simulink model "sequentialProcessorNarenKolli"  (R2018b)
settings: Solver=VariableStepAuto  StartTime=0.0  StopTime=10  RelTol=1e-3
libraries: hdlsllib x172, simulink_extras x9
(part 3 of 4)

== system sequentialProcessorNarenKolli/8-Bit_Processor /8-Bit_Multiplier/First 8-Bit_Adder/Full Adder5 ==
  X : Inport
  Y : Inport  Port=2
  Z : Inport  Port=3
  Half Adder : Subsystem
  Half Adder1 : Subsystem
  OR : Logic  Operator=OR  AllPortsSameDT=off  OutDataTypeStr=boolean
  S : Outport
  C : Outport  Port=2
  wires:
  Half Adder/2(Carry) -> OR/2
  OR/1 -> C/1
  Z/1 -> Half Adder1/2(B)
  X/1 -> Half Adder/1(A)
  Half Adder1/1(Sum) -> S/1
  Half Adder/1(Sum) -> Half Adder1/1(A)
  Y/1 -> Half Adder/2(B)
  Half Adder1/2(Carry) -> OR/1

== system sequentialProcessorNarenKolli/8-Bit_Processor /8-Bit_Multiplier/First 8-Bit_Adder/Full Adder6 ==
  X : Inport
  Y : Inport  Port=2
  Z : Inport  Port=3
  Half Adder : Subsystem
  Half Adder1 : Subsystem
  OR : Logic  Operator=OR  AllPortsSameDT=off  OutDataTypeStr=boolean
  S : Outport
  C : Outport  Port=2
  wires:
  Half Adder/2(Carry) -> OR/2
  OR/1 -> C/1
  Z/1 -> Half Adder1/2(B)
  X/1 -> Half Adder/1(A)
  Half Adder1/1(Sum) -> S/1
  Half Adder/1(Sum) -> Half Adder1/1(A)
  Y/1 -> Half Adder/2(B)
  Half Adder1/2(Carry) -> OR/1

== system sequentialProcessorNarenKolli/8-Bit_Processor /8-Bit_Multiplier/First 8-Bit_Adder/Full Adder7 ==
  X : Inport
  Y : Inport  Port=2
  Z : Inport  Port=3
  Half Adder : Subsystem
  Half Adder1 : Subsystem
  OR : Logic  Operator=OR  AllPortsSameDT=off  OutDataTypeStr=boolean
  S : Outport
  C : Outport  Port=2
  wires:
  Half Adder/2(Carry) -> OR/2
  OR/1 -> C/1
  Z/1 -> Half Adder1/2(B)
  X/1 -> Half Adder/1(A)
  Half Adder1/1(Sum) -> S/1
  Half Adder/1(Sum) -> Half Adder1/1(A)
  Y/1 -> Half Adder/2(B)
  Half Adder1/2(Carry) -> OR/1

== system sequentialProcessorNarenKolli/8-Bit_Processor /8-Bit_Multiplier/First 8-Bit_Adder/Slicer ==
  X : Inport  OutDataTypeStr=uint8  SampleTime=1
  Bit Slice : hdlsllib/Logic and Bit Operations/Bit Slice  lidx=7  ridx=7
  Bit Slice1 : hdlsllib/Logic and Bit Operations/Bit Slice  lidx=6  ridx=6
  Bit Slice2 : hdlsllib/Logic and Bit Operations/Bit Slice  lidx=5  ridx=5
  Bit Slice3 : hdlsllib/Logic and Bit Operations/Bit Slice  lidx=4  ridx=4
  Bit Slice4 : hdlsllib/Logic and Bit Operations/Bit Slice  lidx=3  ridx=3
  Bit Slice5 : hdlsllib/Logic and Bit Operations/Bit Slice  lidx=2  ridx=2
  Bit Slice6 : hdlsllib/Logic and Bit Operations/Bit Slice  lidx=1  ridx=1
  Bit Slice7 : hdlsllib/Logic and Bit Operations/Bit Slice  lidx=0  ridx=0
  Data Type Conversion{,1..7} (8 alike) : DataTypeConversion
  Y7 : Outport
  Y6 : Outport  Port=2
  Y5 : Outport  Port=3
  Y4 : Outport  Port=4
  Y3 : Outport  Port=5
  Y2 : Outport  Port=6
  Y1 : Outport  Port=7
  Y0 : Outport  Port=8
  wires:
  Data Type Conversion4/1 -> Y4/1
  Bit Slice3/1 -> Data Type Conversion4/1
  X/1 -> Bit Slice3/1, Bit Slice2/1, Bit Slice1/1, Bit Slice/1, Bit Slice4/1, Bit Slice5/1, Bit Slice6/1, Bit Slice7/1
  Bit Slice1/1 -> Data Type Conversion6/1
  Data Type Conversion1/1 -> Y1/1
  Bit Slice6/1 -> Data Type Conversion1/1
  Bit Slice5/1 -> Data Type Conversion2/1
  Bit Slice2/1 -> Data Type Conversion5/1
  Data Type Conversion/1 -> Y0/1
  Bit Slice4/1 -> Data Type Conversion3/1
  Bit Slice/1 -> Data Type Conversion7/1
  Data Type Conversion7/1 -> Y7/1
  Bit Slice7/1 -> Data Type Conversion/1
  Data Type Conversion3/1 -> Y3/1
  Data Type Conversion5/1 -> Y5/1
  Data Type Conversion6/1 -> Y6/1
  Data Type Conversion2/1 -> Y2/1

== system sequentialProcessorNarenKolli/8-Bit_Processor /8-Bit_Multiplier/First 8-Bit_Adder/Slicer1 ==
  X : Inport  OutDataTypeStr=uint8  SampleTime=1
  Bit Slice : hdlsllib/Logic and Bit Operations/Bit Slice  lidx=7  ridx=7
  Bit Slice1 : hdlsllib/Logic and Bit Operations/Bit Slice  lidx=6  ridx=6
  Bit Slice2 : hdlsllib/Logic and Bit Operations/Bit Slice  lidx=5  ridx=5
  Bit Slice3 : hdlsllib/Logic and Bit Operations/Bit Slice  lidx=4  ridx=4
  Bit Slice4 : hdlsllib/Logic and Bit Operations/Bit Slice  lidx=3  ridx=3
  Bit Slice5 : hdlsllib/Logic and Bit Operations/Bit Slice  lidx=2  ridx=2
  Bit Slice6 : hdlsllib/Logic and Bit Operations/Bit Slice  lidx=1  ridx=1
  Bit Slice7 : hdlsllib/Logic and Bit Operations/Bit Slice  lidx=0  ridx=0
  Data Type Conversion{,1..7} (8 alike) : DataTypeConversion
  Y7 : Outport
  Y6 : Outport  Port=2
  Y5 : Outport  Port=3
  Y4 : Outport  Port=4
  Y3 : Outport  Port=5
  Y2 : Outport  Port=6
  Y1 : Outport  Port=7
  Y0 : Outport  Port=8
  wires:
  Data Type Conversion4/1 -> Y4/1
  Bit Slice3/1 -> Data Type Conversion4/1
  X/1 -> Bit Slice3/1, Bit Slice2/1, Bit Slice1/1, Bit Slice/1, Bit Slice4/1, Bit Slice5/1, Bit Slice6/1, Bit Slice7/1
  Bit Slice1/1 -> Data Type Conversion6/1
  Data Type Conversion1/1 -> Y1/1
  Bit Slice6/1 -> Data Type Conversion1/1
  Bit Slice5/1 -> Data Type Conversion2/1
  Bit Slice2/1 -> Data Type Conversion5/1
  Data Type Conversion/1 -> Y0/1
  Bit Slice4/1 -> Data Type Conversion3/1
  Bit Slice/1 -> Data Type Conversion7/1
  Data Type Conversion7/1 -> Y7/1
  Bit Slice7/1 -> Data Type Conversion/1
  Data Type Conversion3/1 -> Y3/1
  Data Type Conversion5/1 -> Y5/1
  Data Type Conversion6/1 -> Y6/1
  Data Type Conversion2/1 -> Y2/1

== system sequentialProcessorNarenKolli/8-Bit_Processor /8-Bit_Multiplier/Second 4x4 Multiplier/Full Adder ==
  X : Inport
  Y : Inport  Port=2
  Z : Inport  Port=3
  Half Adder : Subsystem
  Half Adder1 : Subsystem
  OR : Logic  Operator=OR  AllPortsSameDT=off  OutDataTypeStr=boolean
  S : Outport
  C : Outport  Port=2
  wires:
  Half Adder/2(Carry) -> OR/2
  OR/1 -> C/1
  Z/1 -> Half Adder1/2(B)
  X/1 -> Half Adder/1(A)
  Half Adder1/1(Sum) -> S/1
  Half Adder/1(Sum) -> Half Adder1/1(A)
  Y/1 -> Half Adder/2(B)
  Half Adder1/2(Carry) -> OR/1

== system sequentialProcessorNarenKolli/8-Bit_Processor /8-Bit_Multiplier/Second 4x4 Multiplier/Full Adder1 ==
  X : Inport
  Y : Inport  Port=2
  Z : Inport  Port=3
  Half Adder : Subsystem
  Half Adder1 : Subsystem
  OR : Logic  Operator=OR  AllPortsSameDT=off  OutDataTypeStr=boolean
  S : Outport
  C : Outport  Port=2
  wires:
  Half Adder/2(Carry) -> OR/2
  OR/1 -> C/1
  Z/1 -> Half Adder1/2(B)
  X/1 -> Half Adder/1(A)
  Half Adder1/1(Sum) -> S/1
  Half Adder/1(Sum) -> Half Adder1/1(A)
  Y/1 -> Half Adder/2(B)
  Half Adder1/2(Carry) -> OR/1

== system sequentialProcessorNarenKolli/8-Bit_Processor /8-Bit_Multiplier/Second 4x4 Multiplier/Full Adder2 ==
  X : Inport
  Y : Inport  Port=2
  Z : Inport  Port=3
  Half Adder : Subsystem
  Half Adder1 : Subsystem
  OR : Logic  Operator=OR  AllPortsSameDT=off  OutDataTypeStr=boolean
  S : Outport
  C : Outport  Port=2
  wires:
  Half Adder/2(Carry) -> OR/2
  OR/1 -> C/1
  Z/1 -> Half Adder1/2(B)
  X/1 -> Half Adder/1(A)
  Half Adder1/1(Sum) -> S/1
  Half Adder/1(Sum) -> Half Adder1/1(A)
  Y/1 -> Half Adder/2(B)
  Half Adder1/2(Carry) -> OR/1

== system sequentialProcessorNarenKolli/8-Bit_Processor /8-Bit_Multiplier/Second 4x4 Multiplier/Full Adder3 ==
  X : Inport
  Y : Inport  Port=2
  Z : Inport  Port=3
  Half Adder : Subsystem
  Half Adder1 : Subsystem
  OR : Logic  Operator=OR  AllPortsSameDT=off  OutDataTypeStr=boolean
  S : Outport
  C : Outport  Port=2
  wires:
  Half Adder/2(Carry) -> OR/2
  OR/1 -> C/1
  Z/1 -> Half Adder1/2(B)
  X/1 -> Half Adder/1(A)
  Half Adder1/1(Sum) -> S/1
  Half Adder/1(Sum) -> Half Adder1/1(A)
  Y/1 -> Half Adder/2(B)
  Half Adder1/2(Carry) -> OR/1

== system sequentialProcessorNarenKolli/8-Bit_Processor /8-Bit_Multiplier/Second 4x4 Multiplier/Full Adder4 ==
  X : Inport
  Y : Inport  Port=2
  Z : Inport  Port=3
  Half Adder : Subsystem
  Half Adder1 : Subsystem
  OR : Logic  Operator=OR  AllPortsSameDT=off  OutDataTypeStr=boolean
  S : Outport
  C : Outport  Port=2
  wires:
  Half Adder/2(Carry) -> OR/2
  OR/1 -> C/1
  Z/1 -> Half Adder1/2(B)
  X/1 -> Half Adder/1(A)
  Half Adder1/1(Sum) -> S/1
  Half Adder/1(Sum) -> Half Adder1/1(A)
  Y/1 -> Half Adder/2(B)
  Half Adder1/2(Carry) -> OR/1

== system sequentialProcessorNarenKolli/8-Bit_Processor /8-Bit_Multiplier/Second 4x4 Multiplier/Full Adder5 ==
  X : Inport
  Y : Inport  Port=2
  Z : Inport  Port=3
  Half Adder : Subsystem
  Half Adder1 : Subsystem
  OR : Logic  Operator=OR  AllPortsSameDT=off  OutDataTypeStr=boolean
  S : Outport
  C : Outport  Port=2
  wires:
  Half Adder/2(Carry) -> OR/2
  OR/1 -> C/1
  Z/1 -> Half Adder1/2(B)
  X/1 -> Half Adder/1(A)
  Half Adder1/1(Sum) -> S/1
  Half Adder/1(Sum) -> Half Adder1/1(A)
  Y/1 -> Half Adder/2(B)
  Half Adder1/2(Carry) -> OR/1

== system sequentialProcessorNarenKolli/8-Bit_Processor /8-Bit_Multiplier/Second 4x4 Multiplier/Full Adder6 ==
  X : Inport
  Y : Inport  Port=2
  Z : Inport  Port=3
  Half Adder : Subsystem
  Half Adder1 : Subsystem
  OR : Logic  Operator=OR  AllPortsSameDT=off  OutDataTypeStr=boolean
  S : Outport
  C : Outport  Port=2
  wires:
  Half Adder/2(Carry) -> OR/2
  OR/1 -> C/1
  Z/1 -> Half Adder1/2(B)
  X/1 -> Half Adder/1(A)
  Half Adder1/1(Sum) -> S/1
  Half Adder/1(Sum) -> Half Adder1/1(A)
  Y/1 -> Half Adder/2(B)
  Half Adder1/2(Carry) -> OR/1

== system sequentialProcessorNarenKolli/8-Bit_Processor /8-Bit_Multiplier/Second 4x4 Multiplier/Full Adder7 ==
  X : Inport
  Y : Inport  Port=2
  Z : Inport  Port=3
  Half Adder : Subsystem
  Half Adder1 : Subsystem
  OR : Logic  Operator=OR  AllPortsSameDT=off  OutDataTypeStr=boolean
  S : Outport
  C : Outport  Port=2
  wires:
  Half Adder/2(Carry) -> OR/2
  OR/1 -> C/1
  Z/1 -> Half Adder1/2(B)
  X/1 -> Half Adder/1(A)
  Half Adder1/1(Sum) -> S/1
  Half Adder/1(Sum) -> Half Adder1/1(A)
  Y/1 -> Half Adder/2(B)
  Half Adder1/2(Carry) -> OR/1

== system sequentialProcessorNarenKolli/8-Bit_Processor /8-Bit_Multiplier/Second 4x4 Multiplier/Half Adder ==
  A : Inport
  B : Inport  Port=2
  AND (calculates carry) : Logic  AllPortsSameDT=off  OutDataTypeStr=boolean
  XOR (calculates sum) : Logic  Operator=XOR  AllPortsSameDT=off  OutDataTypeStr=boolean
  Sum : Outport
  Carry : Outport  Port=2
  wires:
  XOR (calculates sum)/1 -> Sum/1
  B/1 -> XOR (calculates sum)/2, AND (calculates carry)/2
  A/1 -> AND (calculates carry)/1, XOR (calculates sum)/1
  AND (calculates carry)/1 -> Carry/1

== system sequentialProcessorNarenKolli/8-Bit_Processor /8-Bit_Multiplier/Second 4x4 Multiplier/Half Adder1 ==
  A : Inport
  B : Inport  Port=2
  AND (calculates carry) : Logic  AllPortsSameDT=off  OutDataTypeStr=boolean
  XOR (calculates sum) : Logic  Operator=XOR  AllPortsSameDT=off  OutDataTypeStr=boolean
  Sum : Outport
  Carry : Outport  Port=2
  wires:
  XOR (calculates sum)/1 -> Sum/1
  B/1 -> XOR (calculates sum)/2, AND (calculates carry)/2
  A/1 -> AND (calculates carry)/1, XOR (calculates sum)/1
  AND (calculates carry)/1 -> Carry/1

== system sequentialProcessorNarenKolli/8-Bit_Processor /8-Bit_Multiplier/Second 4x4 Multiplier/Half Adder2 ==
  A : Inport
  B : Inport  Port=2
  AND (calculates carry) : Logic  AllPortsSameDT=off  OutDataTypeStr=boolean
  XOR (calculates sum) : Logic  Operator=XOR  AllPortsSameDT=off  OutDataTypeStr=boolean
  Sum : Outport
  Carry : Outport  Port=2
  wires:
  XOR (calculates sum)/1 -> Sum/1
  B/1 -> XOR (calculates sum)/2, AND (calculates carry)/2
  A/1 -> AND (calculates carry)/1, XOR (calculates sum)/1
  AND (calculates carry)/1 -> Carry/1

== system sequentialProcessorNarenKolli/8-Bit_Processor /8-Bit_Multiplier/Second 4x4 Multiplier/Half Adder3 ==
  A : Inport
  B : Inport  Port=2
  AND (calculates carry) : Logic  AllPortsSameDT=off  OutDataTypeStr=boolean
  XOR (calculates sum) : Logic  Operator=XOR  AllPortsSameDT=off  OutDataTypeStr=boolean
  Sum : Outport
  Carry : Outport  Port=2
  wires:
  XOR (calculates sum)/1 -> Sum/1
  B/1 -> XOR (calculates sum)/2, AND (calculates carry)/2
  A/1 -> AND (calculates carry)/1, XOR (calculates sum)/1
  AND (calculates carry)/1 -> Carry/1

== system sequentialProcessorNarenKolli/8-Bit_Processor /8-Bit_Multiplier/Second 8-Bit_Adder1/Full Adder ==
  X : Inport
  Y : Inport  Port=2
  Z : Inport  Port=3
  Half Adder : Subsystem
  Half Adder1 : Subsystem
  OR : Logic  Operator=OR  AllPortsSameDT=off  OutDataTypeStr=boolean
  S : Outport
  C : Outport  Port=2
  wires:
  Half Adder/2(Carry) -> OR/2
  OR/1 -> C/1
  Z/1 -> Half Adder1/2(B)
  X/1 -> Half Adder/1(A)
  Half Adder1/1(Sum) -> S/1
  Half Adder/1(Sum) -> Half Adder1/1(A)
  Y/1 -> Half Adder/2(B)
  Half Adder1/2(Carry) -> OR/1

== system sequentialProcessorNarenKolli/8-Bit_Processor /8-Bit_Multiplier/Second 8-Bit_Adder1/Full Adder1 ==
  X : Inport
  Y : Inport  Port=2
  Z : Inport  Port=3
  Half Adder : Subsystem
  Half Adder1 : Subsystem
  OR : Logic  Operator=OR  AllPortsSameDT=off  OutDataTypeStr=boolean
  S : Outport
  C : Outport  Port=2
  wires:
  Half Adder/2(Carry) -> OR/2
  OR/1 -> C/1
  Z/1 -> Half Adder1/2(B)
  X/1 -> Half Adder/1(A)
  Half Adder1/1(Sum) -> S/1
  Half Adder/1(Sum) -> Half Adder1/1(A)
  Y/1 -> Half Adder/2(B)
  Half Adder1/2(Carry) -> OR/1

== system sequentialProcessorNarenKolli/8-Bit_Processor /8-Bit_Multiplier/Second 8-Bit_Adder1/Full Adder2 ==
  X : Inport
  Y : Inport  Port=2
  Z : Inport  Port=3
  Half Adder : Subsystem
  Half Adder1 : Subsystem
  OR : Logic  Operator=OR  AllPortsSameDT=off  OutDataTypeStr=boolean
  S : Outport
  C : Outport  Port=2
  wires:
  Half Adder/2(Carry) -> OR/2
  OR/1 -> C/1
  Z/1 -> Half Adder1/2(B)
  X/1 -> Half Adder/1(A)
  Half Adder1/1(Sum) -> S/1
  Half Adder/1(Sum) -> Half Adder1/1(A)
  Y/1 -> Half Adder/2(B)
  Half Adder1/2(Carry) -> OR/1

== system sequentialProcessorNarenKolli/8-Bit_Processor /8-Bit_Multiplier/Second 8-Bit_Adder1/Full Adder3 ==
  X : Inport
  Y : Inport  Port=2
  Z : Inport  Port=3
  Half Adder : Subsystem
  Half Adder1 : Subsystem
  OR : Logic  Operator=OR  AllPortsSameDT=off  OutDataTypeStr=boolean
  S : Outport
  C : Outport  Port=2
  wires:
  Half Adder/2(Carry) -> OR/2
  OR/1 -> C/1
  Z/1 -> Half Adder1/2(B)
  X/1 -> Half Adder/1(A)
  Half Adder1/1(Sum) -> S/1
  Half Adder/1(Sum) -> Half Adder1/1(A)
  Y/1 -> Half Adder/2(B)
  Half Adder1/2(Carry) -> OR/1

== system sequentialProcessorNarenKolli/8-Bit_Processor /8-Bit_Multiplier/Second 8-Bit_Adder1/Full Adder4 ==
  X : Inport
  Y : Inport  Port=2
  Z : Inport  Port=3
  Half Adder : Subsystem
  Half Adder1 : Subsystem
  OR : Logic  Operator=OR  AllPortsSameDT=off  OutDataTypeStr=boolean
  S : Outport
  C : Outport  Port=2
  wires:
  Half Adder/2(Carry) -> OR/2
  OR/1 -> C/1
  Z/1 -> Half Adder1/2(B)
  X/1 -> Half Adder/1(A)
  Half Adder1/1(Sum) -> S/1
  Half Adder/1(Sum) -> Half Adder1/1(A)
  Y/1 -> Half Adder/2(B)
  Half Adder1/2(Carry) -> OR/1

== system sequentialProcessorNarenKolli/8-Bit_Processor /8-Bit_Multiplier/Second 8-Bit_Adder1/Full Adder5 ==
  X : Inport
  Y : Inport  Port=2
  Z : Inport  Port=3
  Half Adder : Subsystem
  Half Adder1 : Subsystem
  OR : Logic  Operator=OR  AllPortsSameDT=off  OutDataTypeStr=boolean
  S : Outport
  C : Outport  Port=2
  wires:
  Half Adder/2(Carry) -> OR/2
  OR/1 -> C/1
  Z/1 -> Half Adder1/2(B)
  X/1 -> Half Adder/1(A)
  Half Adder1/1(Sum) -> S/1
  Half Adder/1(Sum) -> Half Adder1/1(A)
  Y/1 -> Half Adder/2(B)
  Half Adder1/2(Carry) -> OR/1

== system sequentialProcessorNarenKolli/8-Bit_Processor /8-Bit_Multiplier/Second 8-Bit_Adder1/Full Adder6 ==
  X : Inport
  Y : Inport  Port=2
  Z : Inport  Port=3
  Half Adder : Subsystem
  Half Adder1 : Subsystem
  OR : Logic  Operator=OR  AllPortsSameDT=off  OutDataTypeStr=boolean
  S : Outport
  C : Outport  Port=2
  wires:
  Half Adder/2(Carry) -> OR/2
  OR/1 -> C/1
  Z/1 -> Half Adder1/2(B)
  X/1 -> Half Adder/1(A)
  Half Adder1/1(Sum) -> S/1
  Half Adder/1(Sum) -> Half Adder1/1(A)
  Y/1 -> Half Adder/2(B)
  Half Adder1/2(Carry) -> OR/1

== system sequentialProcessorNarenKolli/8-Bit_Processor /8-Bit_Multiplier/Second 8-Bit_Adder1/Full Adder7 ==
  X : Inport
  Y : Inport  Port=2
  Z : Inport  Port=3
  Half Adder : Subsystem
  Half Adder1 : Subsystem
  OR : Logic  Operator=OR  AllPortsSameDT=off  OutDataTypeStr=boolean
  S : Outport
  C : Outport  Port=2
  wires:
  Half Adder/2(Carry) -> OR/2
  OR/1 -> C/1
  Z/1 -> Half Adder1/2(B)
  X/1 -> Half Adder/1(A)
  Half Adder1/1(Sum) -> S/1
  Half Adder/1(Sum) -> Half Adder1/1(A)
  Y/1 -> Half Adder/2(B)
  Half Adder1/2(Carry) -> OR/1

== system sequentialProcessorNarenKolli/8-Bit_Processor /8-Bit_Multiplier/Second 8-Bit_Adder1/Slicer ==
  X : Inport  OutDataTypeStr=uint8  SampleTime=1
  Bit Slice : hdlsllib/Logic and Bit Operations/Bit Slice  lidx=7  ridx=7
  Bit Slice1 : hdlsllib/Logic and Bit Operations/Bit Slice  lidx=6  ridx=6
  Bit Slice2 : hdlsllib/Logic and Bit Operations/Bit Slice  lidx=5  ridx=5
  Bit Slice3 : hdlsllib/Logic and Bit Operations/Bit Slice  lidx=4  ridx=4
  Bit Slice4 : hdlsllib/Logic and Bit Operations/Bit Slice  lidx=3  ridx=3
  Bit Slice5 : hdlsllib/Logic and Bit Operations/Bit Slice  lidx=2  ridx=2
  Bit Slice6 : hdlsllib/Logic and Bit Operations/Bit Slice  lidx=1  ridx=1
  Bit Slice7 : hdlsllib/Logic and Bit Operations/Bit Slice  lidx=0  ridx=0
  Data Type Conversion{,1..7} (8 alike) : DataTypeConversion
  Y7 : Outport
  Y6 : Outport  Port=2
  Y5 : Outport  Port=3
  Y4 : Outport  Port=4
  Y3 : Outport  Port=5
  Y2 : Outport  Port=6
  Y1 : Outport  Port=7
  Y0 : Outport  Port=8
  wires:
  Data Type Conversion4/1 -> Y4/1
  Bit Slice3/1 -> Data Type Conversion4/1
  X/1 -> Bit Slice3/1, Bit Slice2/1, Bit Slice1/1, Bit Slice/1, Bit Slice4/1, Bit Slice5/1, Bit Slice6/1, Bit Slice7/1
  Bit Slice1/1 -> Data Type Conversion6/1
  Data Type Conversion1/1 -> Y1/1
  Bit Slice6/1 -> Data Type Conversion1/1
  Bit Slice5/1 -> Data Type Conversion2/1
  Bit Slice2/1 -> Data Type Conversion5/1
  Data Type Conversion/1 -> Y0/1
  Bit Slice4/1 -> Data Type Conversion3/1
  Bit Slice/1 -> Data Type Conversion7/1
  Data Type Conversion7/1 -> Y7/1
  Bit Slice7/1 -> Data Type Conversion/1
  Data Type Conversion3/1 -> Y3/1
  Data Type Conversion5/1 -> Y5/1
  Data Type Conversion6/1 -> Y6/1
  Data Type Conversion2/1 -> Y2/1

== system sequentialProcessorNarenKolli/8-Bit_Processor /8-Bit_Multiplier/Second 8-Bit_Adder1/Slicer1 ==
  X : Inport  OutDataTypeStr=uint8  SampleTime=1
  Bit Slice : hdlsllib/Logic and Bit Operations/Bit Slice  lidx=7  ridx=7
  Bit Slice1 : hdlsllib/Logic and Bit Operations/Bit Slice  lidx=6  ridx=6
  Bit Slice2 : hdlsllib/Logic and Bit Operations/Bit Slice  lidx=5  ridx=5
  Bit Slice3 : hdlsllib/Logic and Bit Operations/Bit Slice  lidx=4  ridx=4
  Bit Slice4 : hdlsllib/Logic and Bit Operations/Bit Slice  lidx=3  ridx=3
  Bit Slice5 : hdlsllib/Logic and Bit Operations/Bit Slice  lidx=2  ridx=2
  Bit Slice6 : hdlsllib/Logic and Bit Operations/Bit Slice  lidx=1  ridx=1
  Bit Slice7 : hdlsllib/Logic and Bit Operations/Bit Slice  lidx=0  ridx=0
  Data Type Conversion{,1..7} (8 alike) : DataTypeConversion
  Y7 : Outport
  Y6 : Outport  Port=2
  Y5 : Outport  Port=3
  Y4 : Outport  Port=4
  Y3 : Outport  Port=5
  Y2 : Outport  Port=6
  Y1 : Outport  Port=7
  Y0 : Outport  Port=8
  wires:
  Data Type Conversion4/1 -> Y4/1
  Bit Slice3/1 -> Data Type Conversion4/1
  X/1 -> Bit Slice3/1, Bit Slice2/1, Bit Slice1/1, Bit Slice/1, Bit Slice4/1, Bit Slice5/1, Bit Slice6/1, Bit Slice7/1
  Bit Slice1/1 -> Data Type Conversion6/1
  Data Type Conversion1/1 -> Y1/1
  Bit Slice6/1 -> Data Type Conversion1/1
  Bit Slice5/1 -> Data Type Conversion2/1
  Bit Slice2/1 -> Data Type Conversion5/1
  Data Type Conversion/1 -> Y0/1
  Bit Slice4/1 -> Data Type Conversion3/1
  Bit Slice/1 -> Data Type Conversion7/1
  Data Type Conversion7/1 -> Y7/1
  Bit Slice7/1 -> Data Type Conversion/1
  Data Type Conversion3/1 -> Y3/1
  Data Type Conversion5/1 -> Y5/1
  Data Type Conversion6/1 -> Y6/1
  Data Type Conversion2/1 -> Y2/1

== system sequentialProcessorNarenKolli/8-Bit_Processor /8-Bit_Multiplier/Third 4x4 Multiplier/Full Adder ==
  X : Inport
  Y : Inport  Port=2
  Z : Inport  Port=3
  Half Adder : Subsystem
  Half Adder1 : Subsystem
  OR : Logic  Operator=OR  AllPortsSameDT=off  OutDataTypeStr=boolean
  S : Outport
  C : Outport  Port=2
  wires:
  Half Adder/2(Carry) -> OR/2
  OR/1 -> C/1
  Z/1 -> Half Adder1/2(B)
  X/1 -> Half Adder/1(A)
  Half Adder1/1(Sum) -> S/1
  Half Adder/1(Sum) -> Half Adder1/1(A)
  Y/1 -> Half Adder/2(B)
  Half Adder1/2(Carry) -> OR/1

== system sequentialProcessorNarenKolli/8-Bit_Processor /8-Bit_Multiplier/Third 4x4 Multiplier/Full Adder1 ==
  X : Inport
  Y : Inport  Port=2
  Z : Inport  Port=3
  Half Adder : Subsystem
  Half Adder1 : Subsystem
  OR : Logic  Operator=OR  AllPortsSameDT=off  OutDataTypeStr=boolean
  S : Outport
  C : Outport  Port=2
  wires:
  Half Adder/2(Carry) -> OR/2
  OR/1 -> C/1
  Z/1 -> Half Adder1/2(B)
  X/1 -> Half Adder/1(A)
  Half Adder1/1(Sum) -> S/1
  Half Adder/1(Sum) -> Half Adder1/1(A)
  Y/1 -> Half Adder/2(B)
  Half Adder1/2(Carry) -> OR/1

== system sequentialProcessorNarenKolli/8-Bit_Processor /8-Bit_Multiplier/Third 4x4 Multiplier/Full Adder2 ==
  X : Inport
  Y : Inport  Port=2
  Z : Inport  Port=3
  Half Adder : Subsystem
  Half Adder1 : Subsystem
  OR : Logic  Operator=OR  AllPortsSameDT=off  OutDataTypeStr=boolean
  S : Outport
  C : Outport  Port=2
  wires:
  Half Adder/2(Carry) -> OR/2
  OR/1 -> C/1
  Z/1 -> Half Adder1/2(B)
  X/1 -> Half Adder/1(A)
  Half Adder1/1(Sum) -> S/1
  Half Adder/1(Sum) -> Half Adder1/1(A)
  Y/1 -> Half Adder/2(B)
  Half Adder1/2(Carry) -> OR/1

== system sequentialProcessorNarenKolli/8-Bit_Processor /8-Bit_Multiplier/Third 4x4 Multiplier/Full Adder3 ==
  X : Inport
  Y : Inport  Port=2
  Z : Inport  Port=3
  Half Adder : Subsystem
  Half Adder1 : Subsystem
  OR : Logic  Operator=OR  AllPortsSameDT=off  OutDataTypeStr=boolean
  S : Outport
  C : Outport  Port=2
  wires:
  Half Adder/2(Carry) -> OR/2
  OR/1 -> C/1
  Z/1 -> Half Adder1/2(B)
  X/1 -> Half Adder/1(A)
  Half Adder1/1(Sum) -> S/1
  Half Adder/1(Sum) -> Half Adder1/1(A)
  Y/1 -> Half Adder/2(B)
  Half Adder1/2(Carry) -> OR/1

== system sequentialProcessorNarenKolli/8-Bit_Processor /8-Bit_Multiplier/Third 4x4 Multiplier/Full Adder4 ==
  X : Inport
  Y : Inport  Port=2
  Z : Inport  Port=3
  Half Adder : Subsystem
  Half Adder1 : Subsystem
  OR : Logic  Operator=OR  AllPortsSameDT=off  OutDataTypeStr=boolean
  S : Outport
  C : Outport  Port=2
  wires:
  Half Adder/2(Carry) -> OR/2
  OR/1 -> C/1
  Z/1 -> Half Adder1/2(B)
  X/1 -> Half Adder/1(A)
  Half Adder1/1(Sum) -> S/1
  Half Adder/1(Sum) -> Half Adder1/1(A)
  Y/1 -> Half Adder/2(B)
  Half Adder1/2(Carry) -> OR/1

== system sequentialProcessorNarenKolli/8-Bit_Processor /8-Bit_Multiplier/Third 4x4 Multiplier/Full Adder5 ==
  X : Inport
  Y : Inport  Port=2
  Z : Inport  Port=3
  Half Adder : Subsystem
  Half Adder1 : Subsystem
  OR : Logic  Operator=OR  AllPortsSameDT=off  OutDataTypeStr=boolean
  S : Outport
  C : Outport  Port=2
  wires:
  Half Adder/2(Carry) -> OR/2
  OR/1 -> C/1
  Z/1 -> Half Adder1/2(B)
  X/1 -> Half Adder/1(A)
  Half Adder1/1(Sum) -> S/1
  Half Adder/1(Sum) -> Half Adder1/1(A)
  Y/1 -> Half Adder/2(B)
  Half Adder1/2(Carry) -> OR/1

== system sequentialProcessorNarenKolli/8-Bit_Processor /8-Bit_Multiplier/Third 4x4 Multiplier/Full Adder6 ==
  X : Inport
  Y : Inport  Port=2
  Z : Inport  Port=3
  Half Adder : Subsystem
  Half Adder1 : Subsystem
  OR : Logic  Operator=OR  AllPortsSameDT=off  OutDataTypeStr=boolean
  S : Outport
  C : Outport  Port=2
  wires:
  Half Adder/2(Carry) -> OR/2
  OR/1 -> C/1
  Z/1 -> Half Adder1/2(B)
  X/1 -> Half Adder/1(A)
  Half Adder1/1(Sum) -> S/1
  Half Adder/1(Sum) -> Half Adder1/1(A)
  Y/1 -> Half Adder/2(B)
  Half Adder1/2(Carry) -> OR/1

== system sequentialProcessorNarenKolli/8-Bit_Processor /8-Bit_Multiplier/Third 4x4 Multiplier/Full Adder7 ==
  X : Inport
  Y : Inport  Port=2
  Z : Inport  Port=3
  Half Adder : Subsystem
  Half Adder1 : Subsystem
  OR : Logic  Operator=OR  AllPortsSameDT=off  OutDataTypeStr=boolean
  S : Outport
  C : Outport  Port=2
  wires:
  Half Adder/2(Carry) -> OR/2
  OR/1 -> C/1
  Z/1 -> Half Adder1/2(B)
  X/1 -> Half Adder/1(A)
  Half Adder1/1(Sum) -> S/1
  Half Adder/1(Sum) -> Half Adder1/1(A)
  Y/1 -> Half Adder/2(B)
  Half Adder1/2(Carry) -> OR/1

== system sequentialProcessorNarenKolli/8-Bit_Processor /8-Bit_Multiplier/Third 4x4 Multiplier/Half Adder ==
  A : Inport
  B : Inport  Port=2
  AND (calculates carry) : Logic  AllPortsSameDT=off  OutDataTypeStr=boolean
  XOR (calculates sum) : Logic  Operator=XOR  AllPortsSameDT=off  OutDataTypeStr=boolean
  Sum : Outport
  Carry : Outport  Port=2
  wires:
  XOR (calculates sum)/1 -> Sum/1
  B/1 -> XOR (calculates sum)/2, AND (calculates carry)/2
  A/1 -> AND (calculates carry)/1, XOR (calculates sum)/1
  AND (calculates carry)/1 -> Carry/1

== system sequentialProcessorNarenKolli/8-Bit_Processor /8-Bit_Multiplier/Third 4x4 Multiplier/Half Adder1 ==
  A : Inport
  B : Inport  Port=2
  AND (calculates carry) : Logic  AllPortsSameDT=off  OutDataTypeStr=boolean
  XOR (calculates sum) : Logic  Operator=XOR  AllPortsSameDT=off  OutDataTypeStr=boolean
  Sum : Outport
  Carry : Outport  Port=2
  wires:
  XOR (calculates sum)/1 -> Sum/1
  B/1 -> XOR (calculates sum)/2, AND (calculates carry)/2
  A/1 -> AND (calculates carry)/1, XOR (calculates sum)/1
  AND (calculates carry)/1 -> Carry/1

== system sequentialProcessorNarenKolli/8-Bit_Processor /8-Bit_Multiplier/Third 4x4 Multiplier/Half Adder2 ==
  A : Inport
  B : Inport  Port=2
  AND (calculates carry) : Logic  AllPortsSameDT=off  OutDataTypeStr=boolean
  XOR (calculates sum) : Logic  Operator=XOR  AllPortsSameDT=off  OutDataTypeStr=boolean
  Sum : Outport
  Carry : Outport  Port=2
  wires:
  XOR (calculates sum)/1 -> Sum/1
  B/1 -> XOR (calculates sum)/2, AND (calculates carry)/2
  A/1 -> AND (calculates carry)/1, XOR (calculates sum)/1
  AND (calculates carry)/1 -> Carry/1

== system sequentialProcessorNarenKolli/8-Bit_Processor /8-Bit_Multiplier/Third 4x4 Multiplier/Half Adder3 ==
  A : Inport
  B : Inport  Port=2
  AND (calculates carry) : Logic  AllPortsSameDT=off  OutDataTypeStr=boolean
  XOR (calculates sum) : Logic  Operator=XOR  AllPortsSameDT=off  OutDataTypeStr=boolean
  Sum : Outport
  Carry : Outport  Port=2
  wires:
  XOR (calculates sum)/1 -> Sum/1
  B/1 -> XOR (calculates sum)/2, AND (calculates carry)/2
  A/1 -> AND (calculates carry)/1, XOR (calculates sum)/1
  AND (calculates carry)/1 -> Carry/1

== system sequentialProcessorNarenKolli/8-Bit_Processor /8-Bit_Subtractor/Full Adder 0/Half Adder ==
  A : Inport
  B : Inport  Port=2
  AND (calculates carry) : Logic  AllPortsSameDT=off  OutDataTypeStr=boolean
  XOR (calculates sum) : Logic  Operator=XOR  AllPortsSameDT=off  OutDataTypeStr=boolean
  Sum : Outport
  Carry : Outport  Port=2
  wires:
  XOR (calculates sum)/1 -> Sum/1
  B/1 -> XOR (calculates sum)/2, AND (calculates carry)/2
  A/1 -> AND (calculates carry)/1, XOR (calculates sum)/1
  AND (calculates carry)/1 -> Carry/1

== system sequentialProcessorNarenKolli/8-Bit_Processor /8-Bit_Subtractor/Full Adder 0/Half Adder1 ==
  A : Inport
  B : Inport  Port=2
  AND (calculates carry) : Logic  AllPortsSameDT=off  OutDataTypeStr=boolean
  XOR (calculates sum) : Logic  Operator=XOR  AllPortsSameDT=off  OutDataTypeStr=boolean
  Sum : Outport
  Carry : Outport  Port=2
  wires:
  XOR (calculates sum)/1 -> Sum/1
  B/1 -> XOR (calculates sum)/2, AND (calculates carry)/2
  A/1 -> AND (calculates carry)/1, XOR (calculates sum)/1
  AND (calculates carry)/1 -> Carry/1

== system sequentialProcessorNarenKolli/8-Bit_Processor /8-Bit_Subtractor/Full Adder 1/Half Adder ==
  A : Inport
  B : Inport  Port=2
  AND (calculates carry) : Logic  AllPortsSameDT=off  OutDataTypeStr=boolean
  XOR (calculates sum) : Logic  Operator=XOR  AllPortsSameDT=off  OutDataTypeStr=boolean
  Sum : Outport
  Carry : Outport  Port=2
  wires:
  XOR (calculates sum)/1 -> Sum/1
  B/1 -> XOR (calculates sum)/2, AND (calculates carry)/2
  A/1 -> AND (calculates carry)/1, XOR (calculates sum)/1
  AND (calculates carry)/1 -> Carry/1

== system sequentialProcessorNarenKolli/8-Bit_Processor /8-Bit_Subtractor/Full Adder 1/Half Adder1 ==
  A : Inport
  B : Inport  Port=2
  AND (calculates carry) : Logic  AllPortsSameDT=off  OutDataTypeStr=boolean
  XOR (calculates sum) : Logic  Operator=XOR  AllPortsSameDT=off  OutDataTypeStr=boolean
  Sum : Outport
  Carry : Outport  Port=2
  wires:
  XOR (calculates sum)/1 -> Sum/1
  B/1 -> XOR (calculates sum)/2, AND (calculates carry)/2
  A/1 -> AND (calculates carry)/1, XOR (calculates sum)/1
  AND (calculates carry)/1 -> Carry/1

== system sequentialProcessorNarenKolli/8-Bit_Processor /8-Bit_Subtractor/Full Adder 2 /Half Adder ==
  A : Inport
  B : Inport  Port=2
  AND (calculates carry) : Logic  AllPortsSameDT=off  OutDataTypeStr=boolean
  XOR (calculates sum) : Logic  Operator=XOR  AllPortsSameDT=off  OutDataTypeStr=boolean
  Sum : Outport
  Carry : Outport  Port=2
  wires:
  XOR (calculates sum)/1 -> Sum/1
  B/1 -> XOR (calculates sum)/2, AND (calculates carry)/2
  A/1 -> AND (calculates carry)/1, XOR (calculates sum)/1
  AND (calculates carry)/1 -> Carry/1

== system sequentialProcessorNarenKolli/8-Bit_Processor /8-Bit_Subtractor/Full Adder 2 /Half Adder1 ==
  A : Inport
  B : Inport  Port=2
  AND (calculates carry) : Logic  AllPortsSameDT=off  OutDataTypeStr=boolean
  XOR (calculates sum) : Logic  Operator=XOR  AllPortsSameDT=off  OutDataTypeStr=boolean
  Sum : Outport
  Carry : Outport  Port=2
  wires:
  XOR (calculates sum)/1 -> Sum/1
  B/1 -> XOR (calculates sum)/2, AND (calculates carry)/2
  A/1 -> AND (calculates carry)/1, XOR (calculates sum)/1
  AND (calculates carry)/1 -> Carry/1

== system sequentialProcessorNarenKolli/8-Bit_Processor /8-Bit_Subtractor/Full Adder 3 /Half Adder ==
  A : Inport
  B : Inport  Port=2
  AND (calculates carry) : Logic  AllPortsSameDT=off  OutDataTypeStr=boolean
  XOR (calculates sum) : Logic  Operator=XOR  AllPortsSameDT=off  OutDataTypeStr=boolean
  Sum : Outport
  Carry : Outport  Port=2
  wires:
  XOR (calculates sum)/1 -> Sum/1
  B/1 -> XOR (calculates sum)/2, AND (calculates carry)/2
  A/1 -> AND (calculates carry)/1, XOR (calculates sum)/1
  AND (calculates carry)/1 -> Carry/1

== system sequentialProcessorNarenKolli/8-Bit_Processor /8-Bit_Subtractor/Full Adder 3 /Half Adder1 ==
  A : Inport
  B : Inport  Port=2
  AND (calculates carry) : Logic  AllPortsSameDT=off  OutDataTypeStr=boolean
  XOR (calculates sum) : Logic  Operator=XOR  AllPortsSameDT=off  OutDataTypeStr=boolean
  Sum : Outport
  Carry : Outport  Port=2
  wires:
  XOR (calculates sum)/1 -> Sum/1
  B/1 -> XOR (calculates sum)/2, AND (calculates carry)/2
  A/1 -> AND (calculates carry)/1, XOR (calculates sum)/1
  AND (calculates carry)/1 -> Carry/1

== system sequentialProcessorNarenKolli/8-Bit_Processor /8-Bit_Subtractor/Full Adder 4/Half Adder ==
  A : Inport
  B : Inport  Port=2
  AND (calculates carry) : Logic  AllPortsSameDT=off  OutDataTypeStr=boolean
  XOR (calculates sum) : Logic  Operator=XOR  AllPortsSameDT=off  OutDataTypeStr=boolean
  Sum : Outport
  Carry : Outport  Port=2
  wires:
  XOR (calculates sum)/1 -> Sum/1
  B/1 -> XOR (calculates sum)/2, AND (calculates carry)/2
  A/1 -> AND (calculates carry)/1, XOR (calculates sum)/1
  AND (calculates carry)/1 -> Carry/1

== system sequentialProcessorNarenKolli/8-Bit_Processor /8-Bit_Subtractor/Full Adder 4/Half Adder1 ==
  A : Inport
  B : Inport  Port=2
  AND (calculates carry) : Logic  AllPortsSameDT=off  OutDataTypeStr=boolean
  XOR (calculates sum) : Logic  Operator=XOR  AllPortsSameDT=off  OutDataTypeStr=boolean
  Sum : Outport
  Carry : Outport  Port=2
  wires:
  XOR (calculates sum)/1 -> Sum/1
  B/1 -> XOR (calculates sum)/2, AND (calculates carry)/2
  A/1 -> AND (calculates carry)/1, XOR (calculates sum)/1
  AND (calculates carry)/1 -> Carry/1

== system sequentialProcessorNarenKolli/8-Bit_Processor /8-Bit_Subtractor/Full Adder 5 /Half Adder ==
  A : Inport
  B : Inport  Port=2
  AND (calculates carry) : Logic  AllPortsSameDT=off  OutDataTypeStr=boolean
  XOR (calculates sum) : Logic  Operator=XOR  AllPortsSameDT=off  OutDataTypeStr=boolean
  Sum : Outport
  Carry : Outport  Port=2
  wires:
  XOR (calculates sum)/1 -> Sum/1
  B/1 -> XOR (calculates sum)/2, AND (calculates carry)/2
  A/1 -> AND (calculates carry)/1, XOR (calculates sum)/1
  AND (calculates carry)/1 -> Carry/1

== system sequentialProcessorNarenKolli/8-Bit_Processor /8-Bit_Subtractor/Full Adder 5 /Half Adder1 ==
  A : Inport
  B : Inport  Port=2
  AND (calculates carry) : Logic  AllPortsSameDT=off  OutDataTypeStr=boolean
  XOR (calculates sum) : Logic  Operator=XOR  AllPortsSameDT=off  OutDataTypeStr=boolean
  Sum : Outport
  Carry : Outport  Port=2
  wires:
  XOR (calculates sum)/1 -> Sum/1
  B/1 -> XOR (calculates sum)/2, AND (calculates carry)/2
  A/1 -> AND (calculates carry)/1, XOR (calculates sum)/1
  AND (calculates carry)/1 -> Carry/1

== system sequentialProcessorNarenKolli/8-Bit_Processor /8-Bit_Subtractor/Full Adder 6 /Half Adder ==
  A : Inport
  B : Inport  Port=2
  AND (calculates carry) : Logic  AllPortsSameDT=off  OutDataTypeStr=boolean
  XOR (calculates sum) : Logic  Operator=XOR  AllPortsSameDT=off  OutDataTypeStr=boolean
  Sum : Outport
  Carry : Outport  Port=2
  wires:
  XOR (calculates sum)/1 -> Sum/1
  B/1 -> XOR (calculates sum)/2, AND (calculates carry)/2
  A/1 -> AND (calculates carry)/1, XOR (calculates sum)/1
  AND (calculates carry)/1 -> Carry/1

== system sequentialProcessorNarenKolli/8-Bit_Processor /8-Bit_Subtractor/Full Adder 6 /Half Adder1 ==
  A : Inport
  B : Inport  Port=2
  AND (calculates carry) : Logic  AllPortsSameDT=off  OutDataTypeStr=boolean
  XOR (calculates sum) : Logic  Operator=XOR  AllPortsSameDT=off  OutDataTypeStr=boolean
  Sum : Outport
  Carry : Outport  Port=2
  wires:
  XOR (calculates sum)/1 -> Sum/1
  B/1 -> XOR (calculates sum)/2, AND (calculates carry)/2
  A/1 -> AND (calculates carry)/1, XOR (calculates sum)/1
  AND (calculates carry)/1 -> Carry/1

== system sequentialProcessorNarenKolli/8-Bit_Processor /8-Bit_Subtractor/Full Adder 7 /Half Adder ==
  A : Inport
  B : Inport  Port=2
  AND (calculates carry) : Logic  AllPortsSameDT=off  OutDataTypeStr=boolean
  XOR (calculates sum) : Logic  Operator=XOR  AllPortsSameDT=off  OutDataTypeStr=boolean
  Sum : Outport
  Carry : Outport  Port=2
  wires:
  XOR (calculates sum)/1 -> Sum/1
  B/1 -> XOR (calculates sum)/2, AND (calculates carry)/2
  A/1 -> AND (calculates carry)/1, XOR (calculates sum)/1
  AND (calculates carry)/1 -> Carry/1

== system sequentialProcessorNarenKolli/8-Bit_Processor /8-Bit_Subtractor/Full Adder 7 /Half Adder1 ==
  A : Inport
  B : Inport  Port=2
  AND (calculates carry) : Logic  AllPortsSameDT=off  OutDataTypeStr=boolean
  XOR (calculates sum) : Logic  Operator=XOR  AllPortsSameDT=off  OutDataTypeStr=boolean
  Sum : Outport
  Carry : Outport  Port=2
  wires:
  XOR (calculates sum)/1 -> Sum/1
  B/1 -> XOR (calculates sum)/2, AND (calculates carry)/2
  A/1 -> AND (calculates carry)/1, XOR (calculates sum)/1
  AND (calculates carry)/1 -> Carry/1

== system sequentialProcessorNarenKolli/8-Bit_Processor /8-Bit_Multiplier/First 4x4 Multiplier /Full Adder/Half Adder ==
  A : Inport
  B : Inport  Port=2
  AND (calculates carry) : Logic  AllPortsSameDT=off  OutDataTypeStr=boolean
  XOR (calculates sum) : Logic  Operator=XOR  AllPortsSameDT=off  OutDataTypeStr=boolean
  Sum : Outport
  Carry : Outport  Port=2
  wires:
  XOR (calculates sum)/1 -> Sum/1
  B/1 -> XOR (calculates sum)/2, AND (calculates carry)/2
  A/1 -> AND (calculates carry)/1, XOR (calculates sum)/1
  AND (calculates carry)/1 -> Carry/1

== system sequentialProcessorNarenKolli/8-Bit_Processor /8-Bit_Multiplier/First 4x4 Multiplier /Full Adder/Half Adder1 ==
  A : Inport
  B : Inport  Port=2
  AND (calculates carry) : Logic  AllPortsSameDT=off  OutDataTypeStr=boolean
  XOR (calculates sum) : Logic  Operator=XOR  AllPortsSameDT=off  OutDataTypeStr=boolean
  Sum : Outport
  Carry : Outport  Port=2
  wires:
  XOR (calculates sum)/1 -> Sum/1
  B/1 -> XOR (calculates sum)/2, AND (calculates carry)/2
  A/1 -> AND (calculates carry)/1, XOR (calculates sum)/1
  AND (calculates carry)/1 -> Carry/1

== system sequentialProcessorNarenKolli/8-Bit_Processor /8-Bit_Multiplier/First 4x4 Multiplier /Full Adder1/Half Adder ==
  A : Inport
  B : Inport  Port=2
  AND (calculates carry) : Logic  AllPortsSameDT=off  OutDataTypeStr=boolean
  XOR (calculates sum) : Logic  Operator=XOR  AllPortsSameDT=off  OutDataTypeStr=boolean
  Sum : Outport
  Carry : Outport  Port=2
  wires:
  XOR (calculates sum)/1 -> Sum/1
  B/1 -> XOR (calculates sum)/2, AND (calculates carry)/2
  A/1 -> AND (calculates carry)/1, XOR (calculates sum)/1
  AND (calculates carry)/1 -> Carry/1

== system sequentialProcessorNarenKolli/8-Bit_Processor /8-Bit_Multiplier/First 4x4 Multiplier /Full Adder1/Half Adder1 ==
  A : Inport
  B : Inport  Port=2
  AND (calculates carry) : Logic  AllPortsSameDT=off  OutDataTypeStr=boolean
  XOR (calculates sum) : Logic  Operator=XOR  AllPortsSameDT=off  OutDataTypeStr=boolean
  Sum : Outport
  Carry : Outport  Port=2
  wires:
  XOR (calculates sum)/1 -> Sum/1
  B/1 -> XOR (calculates sum)/2, AND (calculates carry)/2
  A/1 -> AND (calculates carry)/1, XOR (calculates sum)/1
  AND (calculates carry)/1 -> Carry/1

== system sequentialProcessorNarenKolli/8-Bit_Processor /8-Bit_Multiplier/First 4x4 Multiplier /Full Adder2/Half Adder ==
  A : Inport
  B : Inport  Port=2
  AND (calculates carry) : Logic  AllPortsSameDT=off  OutDataTypeStr=boolean
  XOR (calculates sum) : Logic  Operator=XOR  AllPortsSameDT=off  OutDataTypeStr=boolean
  Sum : Outport
  Carry : Outport  Port=2
  wires:
  XOR (calculates sum)/1 -> Sum/1
  B/1 -> XOR (calculates sum)/2, AND (calculates carry)/2
  A/1 -> AND (calculates carry)/1, XOR (calculates sum)/1
  AND (calculates carry)/1 -> Carry/1

== system sequentialProcessorNarenKolli/8-Bit_Processor /8-Bit_Multiplier/First 4x4 Multiplier /Full Adder2/Half Adder1 ==
  A : Inport
  B : Inport  Port=2
  AND (calculates carry) : Logic  AllPortsSameDT=off  OutDataTypeStr=boolean
  XOR (calculates sum) : Logic  Operator=XOR  AllPortsSameDT=off  OutDataTypeStr=boolean
  Sum : Outport
  Carry : Outport  Port=2
  wires:
  XOR (calculates sum)/1 -> Sum/1
  B/1 -> XOR (calculates sum)/2, AND (calculates carry)/2
  A/1 -> AND (calculates carry)/1, XOR (calculates sum)/1
  AND (calculates carry)/1 -> Carry/1

== system sequentialProcessorNarenKolli/8-Bit_Processor /8-Bit_Multiplier/First 4x4 Multiplier /Full Adder3/Half Adder ==
  A : Inport
  B : Inport  Port=2
  AND (calculates carry) : Logic  AllPortsSameDT=off  OutDataTypeStr=boolean
  XOR (calculates sum) : Logic  Operator=XOR  AllPortsSameDT=off  OutDataTypeStr=boolean
  Sum : Outport
  Carry : Outport  Port=2
  wires:
  XOR (calculates sum)/1 -> Sum/1
  B/1 -> XOR (calculates sum)/2, AND (calculates carry)/2
  A/1 -> AND (calculates carry)/1, XOR (calculates sum)/1
  AND (calculates carry)/1 -> Carry/1

== system sequentialProcessorNarenKolli/8-Bit_Processor /8-Bit_Multiplier/First 4x4 Multiplier /Full Adder3/Half Adder1 ==
  A : Inport
  B : Inport  Port=2
  AND (calculates carry) : Logic  AllPortsSameDT=off  OutDataTypeStr=boolean
  XOR (calculates sum) : Logic  Operator=XOR  AllPortsSameDT=off  OutDataTypeStr=boolean
  Sum : Outport
  Carry : Outport  Port=2
  wires:
  XOR (calculates sum)/1 -> Sum/1
  B/1 -> XOR (calculates sum)/2, AND (calculates carry)/2
  A/1 -> AND (calculates carry)/1, XOR (calculates sum)/1
  AND (calculates carry)/1 -> Carry/1

== system sequentialProcessorNarenKolli/8-Bit_Processor /8-Bit_Multiplier/First 4x4 Multiplier /Full Adder4/Half Adder ==
  A : Inport
  B : Inport  Port=2
  AND (calculates carry) : Logic  AllPortsSameDT=off  OutDataTypeStr=boolean
  XOR (calculates sum) : Logic  Operator=XOR  AllPortsSameDT=off  OutDataTypeStr=boolean
  Sum : Outport
  Carry : Outport  Port=2
  wires:
  XOR (calculates sum)/1 -> Sum/1
  B/1 -> XOR (calculates sum)/2, AND (calculates carry)/2
  A/1 -> AND (calculates carry)/1, XOR (calculates sum)/1
  AND (calculates carry)/1 -> Carry/1

== system sequentialProcessorNarenKolli/8-Bit_Processor /8-Bit_Multiplier/First 4x4 Multiplier /Full Adder4/Half Adder1 ==
  A : Inport
  B : Inport  Port=2
  AND (calculates carry) : Logic  AllPortsSameDT=off  OutDataTypeStr=boolean
  XOR (calculates sum) : Logic  Operator=XOR  AllPortsSameDT=off  OutDataTypeStr=boolean
  Sum : Outport
  Carry : Outport  Port=2
  wires:
  XOR (calculates sum)/1 -> Sum/1
  B/1 -> XOR (calculates sum)/2, AND (calculates carry)/2
  A/1 -> AND (calculates carry)/1, XOR (calculates sum)/1
  AND (calculates carry)/1 -> Carry/1

== system sequentialProcessorNarenKolli/8-Bit_Processor /8-Bit_Multiplier/First 4x4 Multiplier /Full Adder5/Half Adder ==
  A : Inport
  B : Inport  Port=2
  AND (calculates carry) : Logic  AllPortsSameDT=off  OutDataTypeStr=boolean
  XOR (calculates sum) : Logic  Operator=XOR  AllPortsSameDT=off  OutDataTypeStr=boolean
  Sum : Outport
  Carry : Outport  Port=2
  wires:
  XOR (calculates sum)/1 -> Sum/1
  B/1 -> XOR (calculates sum)/2, AND (calculates carry)/2
  A/1 -> AND (calculates carry)/1, XOR (calculates sum)/1
  AND (calculates carry)/1 -> Carry/1

== system sequentialProcessorNarenKolli/8-Bit_Processor /8-Bit_Multiplier/First 4x4 Multiplier /Full Adder5/Half Adder1 ==
  A : Inport
  B : Inport  Port=2
  AND (calculates carry) : Logic  AllPortsSameDT=off  OutDataTypeStr=boolean
  XOR (calculates sum) : Logic  Operator=XOR  AllPortsSameDT=off  OutDataTypeStr=boolean
  Sum : Outport
  Carry : Outport  Port=2
  wires:
  XOR (calculates sum)/1 -> Sum/1
  B/1 -> XOR (calculates sum)/2, AND (calculates carry)/2
  A/1 -> AND (calculates carry)/1, XOR (calculates sum)/1
  AND (calculates carry)/1 -> Carry/1

== system sequentialProcessorNarenKolli/8-Bit_Processor /8-Bit_Multiplier/First 4x4 Multiplier /Full Adder6/Half Adder ==
  A : Inport
  B : Inport  Port=2
  AND (calculates carry) : Logic  AllPortsSameDT=off  OutDataTypeStr=boolean
  XOR (calculates sum) : Logic  Operator=XOR  AllPortsSameDT=off  OutDataTypeStr=boolean
  Sum : Outport
  Carry : Outport  Port=2
  wires:
  XOR (calculates sum)/1 -> Sum/1
  B/1 -> XOR (calculates sum)/2, AND (calculates carry)/2
  A/1 -> AND (calculates carry)/1, XOR (calculates sum)/1
  AND (calculates carry)/1 -> Carry/1

== system sequentialProcessorNarenKolli/8-Bit_Processor /8-Bit_Multiplier/First 4x4 Multiplier /Full Adder6/Half Adder1 ==
  A : Inport
  B : Inport  Port=2
  AND (calculates carry) : Logic  AllPortsSameDT=off  OutDataTypeStr=boolean
  XOR (calculates sum) : Logic  Operator=XOR  AllPortsSameDT=off  OutDataTypeStr=boolean
  Sum : Outport
  Carry : Outport  Port=2
  wires:
  XOR (calculates sum)/1 -> Sum/1
  B/1 -> XOR (calculates sum)/2, AND (calculates carry)/2
  A/1 -> AND (calculates carry)/1, XOR (calculates sum)/1
  AND (calculates carry)/1 -> Carry/1

== system sequentialProcessorNarenKolli/8-Bit_Processor /8-Bit_Multiplier/First 4x4 Multiplier /Full Adder7/Half Adder ==
  A : Inport
  B : Inport  Port=2
  AND (calculates carry) : Logic  AllPortsSameDT=off  OutDataTypeStr=boolean
  XOR (calculates sum) : Logic  Operator=XOR  AllPortsSameDT=off  OutDataTypeStr=boolean
  Sum : Outport
  Carry : Outport  Port=2
  wires:
  XOR (calculates sum)/1 -> Sum/1
  B/1 -> XOR (calculates sum)/2, AND (calculates carry)/2
  A/1 -> AND (calculates carry)/1, XOR (calculates sum)/1
  AND (calculates carry)/1 -> Carry/1

== system sequentialProcessorNarenKolli/8-Bit_Processor /8-Bit_Multiplier/First 4x4 Multiplier /Full Adder7/Half Adder1 ==
  A : Inport
  B : Inport  Port=2
  AND (calculates carry) : Logic  AllPortsSameDT=off  OutDataTypeStr=boolean
  XOR (calculates sum) : Logic  Operator=XOR  AllPortsSameDT=off  OutDataTypeStr=boolean
  Sum : Outport
  Carry : Outport  Port=2
  wires:
  XOR (calculates sum)/1 -> Sum/1
  B/1 -> XOR (calculates sum)/2, AND (calculates carry)/2
  A/1 -> AND (calculates carry)/1, XOR (calculates sum)/1
  AND (calculates carry)/1 -> Carry/1

== system sequentialProcessorNarenKolli/8-Bit_Processor /8-Bit_Multiplier/First 8-Bit_Adder/Full Adder/Half Adder ==
  A : Inport
  B : Inport  Port=2
  AND (calculates carry) : Logic  AllPortsSameDT=off  OutDataTypeStr=boolean
  XOR (calculates sum) : Logic  Operator=XOR  AllPortsSameDT=off  OutDataTypeStr=boolean
  Sum : Outport
  Carry : Outport  Port=2
  wires:
  XOR (calculates sum)/1 -> Sum/1
  B/1 -> XOR (calculates sum)/2, AND (calculates carry)/2
  A/1 -> AND (calculates carry)/1, XOR (calculates sum)/1
  AND (calculates carry)/1 -> Carry/1

== system sequentialProcessorNarenKolli/8-Bit_Processor /8-Bit_Multiplier/First 8-Bit_Adder/Full Adder/Half Adder1 ==
  A : Inport
  B : Inport  Port=2
  AND (calculates carry) : Logic  AllPortsSameDT=off  OutDataTypeStr=boolean
  XOR (calculates sum) : Logic  Operator=XOR  AllPortsSameDT=off  OutDataTypeStr=boolean
  Sum : Outport
  Carry : Outport  Port=2
  wires:
  XOR (calculates sum)/1 -> Sum/1
  B/1 -> XOR (calculates sum)/2, AND (calculates carry)/2
  A/1 -> AND (calculates carry)/1, XOR (calculates sum)/1
  AND (calculates carry)/1 -> Carry/1

== system sequentialProcessorNarenKolli/8-Bit_Processor /8-Bit_Multiplier/First 8-Bit_Adder/Full Adder1/Half Adder ==
  A : Inport
  B : Inport  Port=2
  AND (calculates carry) : Logic  AllPortsSameDT=off  OutDataTypeStr=boolean
  XOR (calculates sum) : Logic  Operator=XOR  AllPortsSameDT=off  OutDataTypeStr=boolean
  Sum : Outport
  Carry : Outport  Port=2
  wires:
  XOR (calculates sum)/1 -> Sum/1
  B/1 -> XOR (calculates sum)/2, AND (calculates carry)/2
  A/1 -> AND (calculates carry)/1, XOR (calculates sum)/1
  AND (calculates carry)/1 -> Carry/1

== system sequentialProcessorNarenKolli/8-Bit_Processor /8-Bit_Multiplier/First 8-Bit_Adder/Full Adder1/Half Adder1 ==
  A : Inport
  B : Inport  Port=2
  AND (calculates carry) : Logic  AllPortsSameDT=off  OutDataTypeStr=boolean
  XOR (calculates sum) : Logic  Operator=XOR  AllPortsSameDT=off  OutDataTypeStr=boolean
  Sum : Outport
  Carry : Outport  Port=2
  wires:
  XOR (calculates sum)/1 -> Sum/1
  B/1 -> XOR (calculates sum)/2, AND (calculates carry)/2
  A/1 -> AND (calculates carry)/1, XOR (calculates sum)/1
  AND (calculates carry)/1 -> Carry/1

== system sequentialProcessorNarenKolli/8-Bit_Processor /8-Bit_Multiplier/First 8-Bit_Adder/Full Adder2/Half Adder ==
  A : Inport
  B : Inport  Port=2
  AND (calculates carry) : Logic  AllPortsSameDT=off  OutDataTypeStr=boolean
  XOR (calculates sum) : Logic  Operator=XOR  AllPortsSameDT=off  OutDataTypeStr=boolean
  Sum : Outport
  Carry : Outport  Port=2
  wires:
  XOR (calculates sum)/1 -> Sum/1
  B/1 -> XOR (calculates sum)/2, AND (calculates carry)/2
  A/1 -> AND (calculates carry)/1, XOR (calculates sum)/1
  AND (calculates carry)/1 -> Carry/1

== system sequentialProcessorNarenKolli/8-Bit_Processor /8-Bit_Multiplier/First 8-Bit_Adder/Full Adder2/Half Adder1 ==
  A : Inport
  B : Inport  Port=2
  AND (calculates carry) : Logic  AllPortsSameDT=off  OutDataTypeStr=boolean
  XOR (calculates sum) : Logic  Operator=XOR  AllPortsSameDT=off  OutDataTypeStr=boolean
  Sum : Outport
  Carry : Outport  Port=2
  wires:
  XOR (calculates sum)/1 -> Sum/1
  B/1 -> XOR (calculates sum)/2, AND (calculates carry)/2
  A/1 -> AND (calculates carry)/1, XOR (calculates sum)/1
  AND (calculates carry)/1 -> Carry/1

== system sequentialProcessorNarenKolli/8-Bit_Processor /8-Bit_Multiplier/First 8-Bit_Adder/Full Adder3/Half Adder ==
  A : Inport
  B : Inport  Port=2
  AND (calculates carry) : Logic  AllPortsSameDT=off  OutDataTypeStr=boolean
  XOR (calculates sum) : Logic  Operator=XOR  AllPortsSameDT=off  OutDataTypeStr=boolean
  Sum : Outport
  Carry : Outport  Port=2
  wires:
  XOR (calculates sum)/1 -> Sum/1
  B/1 -> XOR (calculates sum)/2, AND (calculates carry)/2
  A/1 -> AND (calculates carry)/1, XOR (calculates sum)/1
  AND (calculates carry)/1 -> Carry/1

== system sequentialProcessorNarenKolli/8-Bit_Processor /8-Bit_Multiplier/First 8-Bit_Adder/Full Adder3/Half Adder1 ==
  A : Inport
  B : Inport  Port=2
  AND (calculates carry) : Logic  AllPortsSameDT=off  OutDataTypeStr=boolean
  XOR (calculates sum) : Logic  Operator=XOR  AllPortsSameDT=off  OutDataTypeStr=boolean
  Sum : Outport
  Carry : Outport  Port=2
  wires:
  XOR (calculates sum)/1 -> Sum/1
  B/1 -> XOR (calculates sum)/2, AND (calculates carry)/2
  A/1 -> AND (calculates carry)/1, XOR (calculates sum)/1
  AND (calculates carry)/1 -> Carry/1

== system sequentialProcessorNarenKolli/8-Bit_Processor /8-Bit_Multiplier/First 8-Bit_Adder/Full Adder4/Half Adder ==
  A : Inport
  B : Inport  Port=2
  AND (calculates carry) : Logic  AllPortsSameDT=off  OutDataTypeStr=boolean
  XOR (calculates sum) : Logic  Operator=XOR  AllPortsSameDT=off  OutDataTypeStr=boolean
  Sum : Outport
  Carry : Outport  Port=2
  wires:
  XOR (calculates sum)/1 -> Sum/1
  B/1 -> XOR (calculates sum)/2, AND (calculates carry)/2
  A/1 -> AND (calculates carry)/1, XOR (calculates sum)/1
  AND (calculates carry)/1 -> Carry/1

== system sequentialProcessorNarenKolli/8-Bit_Processor /8-Bit_Multiplier/First 8-Bit_Adder/Full Adder4/Half Adder1 ==
  A : Inport
  B : Inport  Port=2
  AND (calculates carry) : Logic  AllPortsSameDT=off  OutDataTypeStr=boolean
  XOR (calculates sum) : Logic  Operator=XOR  AllPortsSameDT=off  OutDataTypeStr=boolean
  Sum : Outport
  Carry : Outport  Port=2
  wires:
  XOR (calculates sum)/1 -> Sum/1
  B/1 -> XOR (calculates sum)/2, AND (calculates carry)/2
  A/1 -> AND (calculates carry)/1, XOR (calculates sum)/1
  AND (calculates carry)/1 -> Carry/1
